simulink model "SoRo_Compliant_Demo_0906"  (R2023b)
settings: Solver=FixedStepAuto  StartTime=0.0  StopTime=inf  FixedStep=0.01  RelTol=1e-3
undefined symbols (not defined in the file): Down, Pull
libraries: simulink x50, speedgoatlib_IO691 x20, canmsglib x19, slpidlib x12, dspfdesign x6
(part 2 of 3)

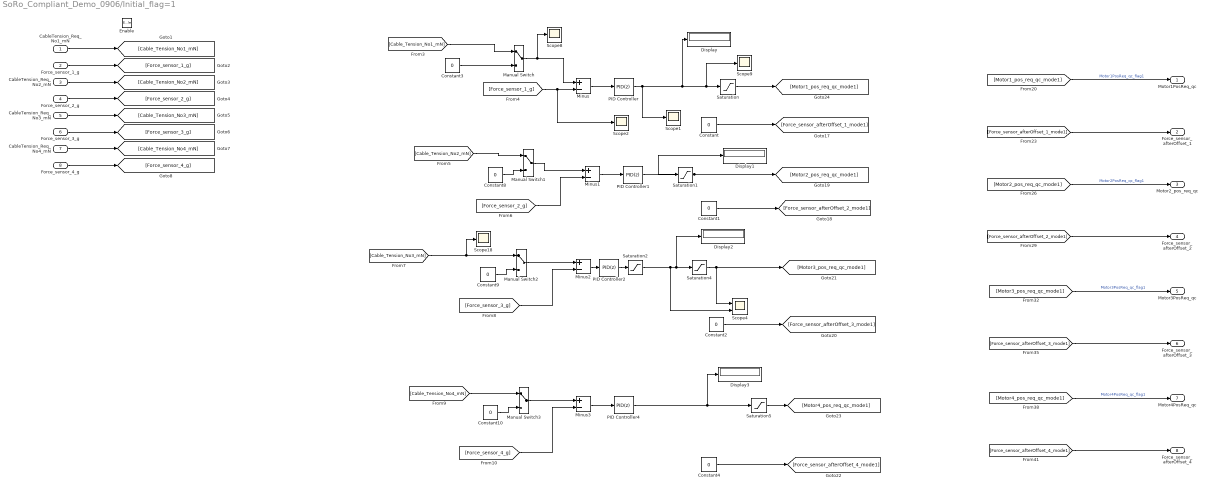
== system SoRo_Compliant_Demo_0906/Initial_flag=1 ==
  CableTension_Req_No1_mN : Inport
  Force_sensor_1_g : Inport  Port=2
  CableTension_Req_No2_mN : Inport  Port=3
  Force_sensor_2_g : Inport  Port=4
  CableTension_Req_No3_mN : Inport  Port=5
  Force_sensor_3_g : Inport  Port=6
  CableTension_Req_No4_mN : Inport  Port=7
  Force_sensor_4_g : Inport  Port=8
  Enable : EnablePort
  Constant{,1..2,4} (4 alike) : Constant  Value=0
  Constant{3,8..10} (4 alike) : Constant  Value=0  SampleTime=0.01
  Display{,1..3} (4 alike) : Display
  Manual Switch{,1..3} (4 alike) : ManualSwitch
  Minus{,1..3} (4 alike) : Sum  Inputs=+-
  PID Controller{,1..2,4} (4 alike) : slpidlib/PID Controller  Controller=PID  Form=Parallel  TimeDomain=Discrete-time  UseExternalTs=off  SampleTime=-1  IntegratorMethod=Forward Euler  FilterMethod=Forward Euler  ControllerParametersSource=internal  P=0.08  I=0.004  UseKiTs=off  D=0  N=100  UseFilter=on  TunerSelectOption=Transfer Function Based (PID Tuner App)  InitialConditionSource=internal  InitialConditionForIntegrator=0  InitialConditionForFilter=0  DifferentiatorICPrevScaledInput=0  ExternalReset=none  TrackingMode=off  Kt=1  LimitOutput=off  SatLimitsSource=internal  UpperSaturationLimit=inf  LowerSaturationLimit=-inf  LinearizeAsGain=on  AntiWindupMode=none  Kb=1  LimitIntegrator=off  UpperIntegratorSaturationLimit=inf  LowerIntegratorSaturationLimit=-inf  POutMin=[]  POutMax=[]  IOutMin=[]  IOutMax=[]  DOutMin=[]  DOutMax=[]  NOutMin=[]  NOutMax=[]  SumOutMin=[]  SumOutMax=[]  SaturationOutMin=[]  SaturationOutMax=[]  PParamMin=[]  PParamMax=[]  IParamMin=[]  IParamMax=[]  DParamMin=[]  DParamMax=[]  NParamMin=[]  NParamMax=[]  KbParamMin=[]  KbParamMax=[]  KtParamMin=[]  KtParamMax=[]  KbOutMin=[]  KbOutMax=[]  KtOutMin=[]  KtOutMax=[]  IntegratorOutMin=[]  IntegratorOutMax=[]  FilterOutMin=[]  FilterOutMax=[]  SumI1OutMin=[]  SumI1OutMax=[]  SumI2OutMin=[]  SumI2OutMax=[]  SumI3OutMin=[]  SumI3OutMax=[]  SumI4OutMin=[]  SumI4OutMax=[]  SumDOutMin=[]  SumDOutMax=[]  DifferentiatorOutMin=[]  DifferentiatorOutMax=[]  FilterDiffOutCoefMin=[]  FilterDiffOutCoefMax=[]  ReciprocalOutMin=[]  ReciprocalOutMax=[]  SumDenOutMin=[]  SumDenOutMax=[]  SumNumOutMin=[]  SumNumOutMax=[]  DivideOutMin=[]  DivideOutMax=[]  UdiffTsProdOutMin=[]  UdiffTsProdOutMax=[]  NTsProdOutMin=[]  NTsProdOutMax=[]  UintegralTsProdOutMin=[]  UintegralTsProdOutMax=[]  UngainTsProdOutMin=[]  UngainTsProdOutMax=[]  ClampingZeroOutDataTypeStr=Inherit: Inherit via back propagation  ClampingZeroOutMin=[]  ClampingZeroOutMax=[]  FilterDenConstantOutDataTypeStr=Inherit: Inherit via back propagation  FilterDenConstantOutMin=[]  FilterDenConstantOutMax=[]  PCopyOutDataTypeStr=Inherit: Inherit via back propagation  PCopyOutMin=[]  PCopyOutMax=[]  NCopyOutDataTypeStr=Inherit: Inherit via back propagation  NCopyOutMin=[]  NCopyOutMax=[]  IntegratorContinuousStateAttributes=''  IntegratorStateMustResolveToSignalObject=off  IntegratorRTWStateStorageClass=Auto  FilterContinuousStateAttributes=''  FilterStateMustResolveToSignalObject=off  FilterRTWStateStorageClass=Auto  ParallelPVariant=InternalParameters  IdealPVariant=Disabled  IVariant=InternalParameters  DVariant=InternalParameters  IntegratorVariant=Discrete  SatVariant=Disabled  AWVariant=Passthrough  PCopyVariant=Disabled  TRVariant=Disabled  FdbkBlocksVariant=Forward  IdealPFdbkVariant=Disabled  SatFdbkVariant=Disabled  DerivativeFilterVariant=ForwardEulerFilter  NVariant=InternalParameters  NCopyVariant=Disabled  FilterICVariant=InternalICsFilter  IntegratorICVariant=InternalICs  ExternalResetVariant=Disabled  TRSumVariant=Passthrough  SumFdbkVariant=Disabled  SumVariant=Sum_PID  TsampFilterVariant=InternalTs  TsampNgainVariant=Passthrough  TsampIntegralVariant=Disabled_SignalSpec  ExternalSaturationOutDataTypeStr=Inherit: Same as second input
  Saturation{,1,4..5} (4 alike) : Saturate  UpperLimit=3000  LowerLimit=-3000
  Saturation2 : Saturate  UpperLimit=400  LowerLimit=-400
  Scope{1..2,8..9,18} (5 alike) : Scope
  Scope4 : Scope  NumInputPorts=2
  Motor1PosReq_qc : Outport
  Force_sensor_afterOffset_1 : Outport  Port=2
  Motor2_pos_req_qc : Outport  Port=3
  Force_sensor_afterOffset_2 : Outport  Port=4
  Motor3PosReq_qc : Outport  Port=5
  Force_sensor_afterOffset_3 : Outport  Port=6
  Motor4PosReq_qc : Outport  Port=7
  Force_sensor_afterOffset_4 : Outport  Port=8
  wires:
  [Force_sensor_afterOffset_4_mode1] -> Force_sensor_afterOffset_4/1
  [Cable_Tension_No1_mN] -> Manual Switch/1
  [Cable_Tension_No4_mN] -> Manual Switch3/1
  Saturation/1 -> [Motor1_pos_req_qc_mode1]
  Constant1/1 -> [Force_sensor_afterOffset_2_mode1]
  [Force_sensor_afterOffset_2_mode1] -> Force_sensor_afterOffset_2/1
  PID Controller4/1 -> Display3/1, Saturation5/1
  PID Controller2/1 -> Saturation2/1
  Manual Switch2/1 -> Minus2/1
  [Cable_Tension_No3_mN] -> Scope18/1, Manual Switch2/1
  PID Controller/1 -> Display/1, Scope9/1, Saturation/1, Scope1/1
  Constant10/1 -> Manual Switch3/2
  Manual Switch3/1 -> Minus3/1
  Manual Switch/1 -> Scope8/1, Minus/1
  Manual Switch1/1 -> Minus1/1
  [Force_sensor_4_g] -> Minus3/2
  [Force_sensor_1_g] -> Scope2/1, Minus/2
  Constant4/1 -> [Force_sensor_afterOffset_4_mode1]
  Constant8/1 -> Manual Switch1/2
  [Cable_Tension_No2_mN] -> Manual Switch1/1
  Constant9/1 -> Manual Switch2/2
  [Force_sensor_2_g] -> Minus1/2
  CableTension_Req_No2_mN/1 -> [Cable_Tension_No2_mN]
  Minus1/1 -> PID Controller1/1
  CableTension_Req_No3_mN/1 -> [Cable_Tension_No3_mN]
  Saturation4/1 -> Scope4/1, [Motor3_pos_req_qc_mode1]
  PID Controller1/1 -> Saturation1/1
  [Force_sensor_afterOffset_3_mode1] -> Force_sensor_afterOffset_3/1
  Minus2/1 -> PID Controller2/1
  Minus/1 -> PID Controller/1
  Force_sensor_3_g/1 -> [Force_sensor_3_g]
  Minus3/1 -> PID Controller4/1
  Saturation2/1 -> Display2/1, Saturation4/1, Scope4/2
  Force_sensor_4_g/1 -> [Force_sensor_4_g]
  CableTension_Req_No4_mN/1 -> [Cable_Tension_No4_mN]
  [Motor4_pos_req_qc_mode1] -> Motor4PosReq_qc/1  "Motor4PosReq_qc_flag1"
  CableTension_Req_No1_mN/1 -> [Cable_Tension_No1_mN]
  Force_sensor_2_g/1 -> [Force_sensor_2_g]
  [Force_sensor_3_g] -> Minus2/2
  [Motor2_pos_req_qc_mode1] -> Motor2_pos_req_qc/1  "Motor2PosReq_qc_flag1"
  Force_sensor_1_g/1 -> [Force_sensor_1_g]
  [Motor3_pos_req_qc_mode1] -> Motor3PosReq_qc/1  "Motor3PosReq_qc_flag1"
  Constant2/1 -> [Force_sensor_afterOffset_3_mode1]
  [Motor1_pos_req_qc_mode1] -> Motor1PosReq_qc/1  "Motor1PosReq_qc_flag1"
  Saturation1/1 -> [Motor2_pos_req_qc_mode1], Display1/1
  Constant3/1 -> Manual Switch/2
  Constant/1 -> [Force_sensor_afterOffset_1_mode1]
  [Force_sensor_afterOffset_1_mode1] -> Force_sensor_afterOffset_1/1
  Saturation5/1 -> [Motor4_pos_req_qc_mode1]

== system SoRo_Compliant_Demo_0906/Subsystem ==
  Channel4 : Inport
  Enable : EnablePort
  " " : Constant  Value=5
  Gain4 : Gain  Gain=0.009
  MATLAB Function4 : MATLAB Function  TreatAsAtomicUnit=on
  MATLAB Function5 : MATLAB Function  TreatAsAtomicUnit=on
  Memory1 : Memory
  Minus2 : Sum  Inputs=+-
  Output Value at Neutral Position : Constant  Value=1000
  Scope{,1..3} (4 alike) : Scope
  Motor5PosReq_qc : Outport
  wires:
  Output Value at Neutral Position/1 -> Minus2/2
  MATLAB Function5/1(y) -> Scope1/1, Minus2/1
  Channel4/1 -> MATLAB Function5/1(u)
  " "/1 -> MATLAB Function5/2(threshold)
  Gain4/1 -> Scope3/1, MATLAB Function4/2(inc)
  Minus2/1 -> Scope2/1, Gain4/1
  Memory1/1 -> MATLAB Function4/1(otpt_last)
  MATLAB Function4/1(y) -> Scope/1, Memory1/1, Motor5PosReq_qc/1  "Motor5PosReq_qc"

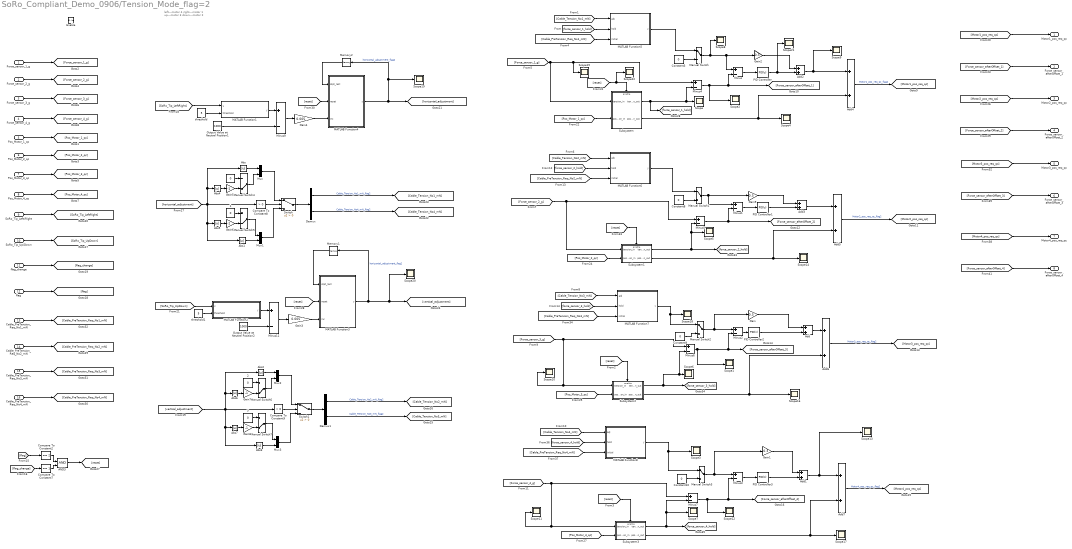
== system SoRo_Compliant_Demo_0906/Tension_Mode_flag=2 ==
  note: left---motor 4
      | right---motor 1
      | up---motor 3
      | down---motor 2
  Force_sensor_1_g : Inport
  Force_sensor_2_g : Inport  Port=2
  Force_sensor_3_g : Inport  Port=3
  Force_sensor_4_g : Inport  Port=4
  Pos_Motor_1_qc : Inport  Port=5
  Pos_Motor_2_qc : Inport  Port=6
  Pos_Motor_3_qc : Inport  Port=7
  Pos_Motor_4_qc : Inport  Port=8
  SoRo_Tip_Left/Right : Inport  Port=9
  SoRo_Tip_Up/Down : Inport  Port=10
  flag_change : Inport  Port=11
  flag : Inport  Port=12
  Cable_PreTension_Req_No1_mN : Inport  Port=13
  Cable_PreTension_Req_No2_mN : Inport  Port=14
  Cable_PreTension_Req_No3_mN : Inport  Port=15
  Cable_PreTension_Req_No4_mN : Inport  Port=16
  Enable : EnablePort
   {,1..3} (4 alike) : Constant  Value=0
  AND3 : Logic  IconShape=distinctive  AllPortsSameDT=off  OutDataTypeStr=boolean
  Abs{,1..7} (8 alike) : Abs  SaturateOnIntegerOverflow=off
  Add{,1..7} (8 alike) : Sum
  Compare To Constant2 : simulink/Logic and Bit Operations/Compare To Constant  relop===  const=2  OutDataTypeStr=boolean
  Compare To Constant7 : simulink/Logic and Bit Operations/Compare To Constant  relop===  const=1  OutDataTypeStr=boolean
  Compare To Constant8 : simulink/Logic and Bit Operations/Compare To Constant  relop=>  const=0  OutDataTypeStr=boolean
  Compare To Constant9 : simulink/Logic and Bit Operations/Compare To Constant  relop=>  const=0  OutDataTypeStr=boolean
  Constant{3,8..10} (4 alike) : Constant  Value=0  SampleTime=0.01
  Demux : Demux  Outputs=2
  Demux1 : Demux  Outputs=2
  Gain{,1..2,9} (4 alike) : Gain  Gain=0.3
  Gain3 : Gain  Gain=0.005
  Gain4 : Gain  Gain=0.005
  Gain{5..8} (4 alike) : Gain  Gain=-1
  MATLAB Function1 : MATLAB Function  TreatAsAtomicUnit=on
  MATLAB Function2 : MATLAB Function  TreatAsAtomicUnit=on
  MATLAB Function3 : MATLAB Function  TreatAsAtomicUnit=on
  MATLAB Function4 : MATLAB Function  TreatAsAtomicUnit=on
  MATLAB Function5 : MATLAB Function  TreatAsAtomicUnit=on
  MATLAB Function6 : MATLAB Function  TreatAsAtomicUnit=on
  MATLAB Function7 : MATLAB Function  TreatAsAtomicUnit=on
  MATLAB Function8 : MATLAB Function  TreatAsAtomicUnit=on
  Manual Switch{,1..3} (4 alike) : ManualSwitch
  Manual Switch{4..7} (4 alike) : ManualSwitch  CurrentSetting=0
  Memory1 : Memory
  Memory2 : Memory
  Minus{,1..7,9,11} (10 alike) : Sum  Inputs=+-
  Mux{,1..3} (4 alike) : Mux  Inputs=2
  Output Value at Neutral Position1 : Constant  Value=1000
  Output Value at Neutral Position2 : Constant  Value=1000
  PID Controller{,1..3} (4 alike) : slpidlib/PID Controller  Controller=PID  Form=Parallel  TimeDomain=Discrete-time  UseExternalTs=off  SampleTime=-1  IntegratorMethod=Forward Euler  FilterMethod=Forward Euler  ControllerParametersSource=internal  P=0.1  I=0  UseKiTs=off  D=0  N=100  UseFilter=on  TunerSelectOption=Transfer Function Based (PID Tuner App)  InitialConditionSource=internal  InitialConditionForIntegrator=0  InitialConditionForFilter=0  DifferentiatorICPrevScaledInput=0  ExternalReset=none  TrackingMode=off  Kt=1  LimitOutput=off  SatLimitsSource=internal  UpperSaturationLimit=inf  LowerSaturationLimit=-inf  LinearizeAsGain=on  AntiWindupMode=none  Kb=1  LimitIntegrator=off  UpperIntegratorSaturationLimit=inf  LowerIntegratorSaturationLimit=-inf  POutMin=[]  POutMax=[]  IOutMin=[]  IOutMax=[]  DOutMin=[]  DOutMax=[]  NOutMin=[]  NOutMax=[]  SumOutMin=[]  SumOutMax=[]  SaturationOutMin=[]  SaturationOutMax=[]  PParamMin=[]  PParamMax=[]  IParamMin=[]  IParamMax=[]  DParamMin=[]  DParamMax=[]  NParamMin=[]  NParamMax=[]  KbParamMin=[]  KbParamMax=[]  KtParamMin=[]  KtParamMax=[]  KbOutMin=[]  KbOutMax=[]  KtOutMin=[]  KtOutMax=[]  IntegratorOutMin=[]  IntegratorOutMax=[]  FilterOutMin=[]  FilterOutMax=[]  SumI1OutMin=[]  SumI1OutMax=[]  SumI2OutMin=[]  SumI2OutMax=[]  SumI3OutMin=[]  SumI3OutMax=[]  SumI4OutMin=[]  SumI4OutMax=[]  SumDOutMin=[]  SumDOutMax=[]  DifferentiatorOutMin=[]  DifferentiatorOutMax=[]  FilterDiffOutCoefMin=[]  FilterDiffOutCoefMax=[]  ReciprocalOutMin=[]  ReciprocalOutMax=[]  SumDenOutMin=[]  SumDenOutMax=[]  SumNumOutMin=[]  SumNumOutMax=[]  DivideOutMin=[]  DivideOutMax=[]  UdiffTsProdOutMin=[]  UdiffTsProdOutMax=[]  NTsProdOutMin=[]  NTsProdOutMax=[]  UintegralTsProdOutMin=[]  UintegralTsProdOutMax=[]  UngainTsProdOutMin=[]  UngainTsProdOutMax=[]  ClampingZeroOutDataTypeStr=Inherit: Inherit via back propagation  ClampingZeroOutMin=[]  ClampingZeroOutMax=[]  FilterDenConstantOutDataTypeStr=Inherit: Inherit via back propagation  FilterDenConstantOutMin=[]  FilterDenConstantOutMax=[]  PCopyOutDataTypeStr=Inherit: Inherit via back propagation  PCopyOutMin=[]  PCopyOutMax=[]  NCopyOutDataTypeStr=Inherit: Inherit via back propagation  NCopyOutMin=[]  NCopyOutMax=[]  IntegratorContinuousStateAttributes=''  IntegratorStateMustResolveToSignalObject=off  IntegratorRTWStateStorageClass=Auto  FilterContinuousStateAttributes=''  FilterStateMustResolveToSignalObject=off  FilterRTWStateStorageClass=Auto  ParallelPVariant=InternalParameters  IdealPVariant=Disabled  IVariant=InternalParameters  DVariant=InternalParameters  IntegratorVariant=Discrete  SatVariant=Disabled  AWVariant=Passthrough  PCopyVariant=Disabled  TRVariant=Disabled  FdbkBlocksVariant=Forward  IdealPFdbkVariant=Disabled  SatFdbkVariant=Disabled  DerivativeFilterVariant=ForwardEulerFilter  NVariant=InternalParameters  NCopyVariant=Disabled  FilterICVariant=InternalICsFilter  IntegratorICVariant=InternalICs  ExternalResetVariant=Disabled  TRSumVariant=Passthrough  SumFdbkVariant=Disabled  SumVariant=Sum_PID  TsampFilterVariant=InternalTs  TsampNgainVariant=Passthrough  TsampIntegralVariant=Disabled_SignalSpec  ExternalSaturationOutDataTypeStr=Inherit: Same as second input
  Scope{,1..22} (23 alike) : Scope
  Subsystem : Subsystem
  Subsystem1 : Subsystem
  Subsystem2 : Subsystem
  Subsystem3 : Subsystem
  Switch : Switch  Criteria=u2 > Threshold  SaturateOnIntegerOverflow=off  InputSameDT=off
  Switch1 : Switch  Criteria=u2 > Threshold  SaturateOnIntegerOverflow=off  InputSameDT=off
  threshold : Constant  Value=5
  threshold1 : Constant  Value=5
  Motor1_pos_req_qc : Outport
  Force_sensor_afterOffset_1 : Outport  Port=2
  Motor2_pos_req_qc : Outport  Port=3
  Force_sensor_afterOffset_2 : Outport  Port=4
  Motor3_pos_req_qc : Outport  Port=5
  Force_sensor_afterOffset_3 : Outport  Port=6
  Motor4_pos_req_qc : Outport  Port=7
  Force_sensor_afterOffset_4 : Outport  Port=8
  wires:
  [Force_sensor_1_g] -> Minus4/1, Scope15/1, Subsystem/1(tension_in)
  [Force_sensor_afterOffset_3] -> Force_sensor_afterOffset_3/1
  [Motor4_pos_req_qc] -> Motor4_pos_req_qc/1
  [Motor1_pos_req_qc] -> Motor1_pos_req_qc/1
  [Force_sensor_afterOffset_4] -> Force_sensor_afterOffset_4/1
  Constant9/1 -> Manual Switch2/2
  Subsystem2/1(tension_out) -> Minus6/2, Scope6/1, [force_sensor_3_hold]
  Minus/1 -> PID Controller/1
  Constant8/1 -> Manual Switch1/2
  [Motor3_pos_req_qc] -> Motor3_pos_req_qc/1
  Add1/1 -> Add7/1, Scope13/1
  Minus1/1 -> PID Controller1/1
  Subsystem3/1(tension_out) -> Scope7/1, Minus7/2, [force_sensor_4_hold]
  Minus7/1 -> Scope12/1, [Force_sensor_afterOffset_4], Minus3/2
  Manual Switch3/1 -> Minus3/1, Gain1/1
  [reset] -> Subsystem1/Enable
  PID Controller2/1 -> Add/2
  Minus5/1 -> [Force_sensor_afterOffset_2], Minus1/2
  Minus6/1 -> Scope1/1, [Force_sensor_afterOffset_3], Minus2/2
  Minus3/1 -> PID Controller3/1
  [Force_sensor_3_g] -> Minus6/1, Subsystem2/1(tension_in), Scope10/1
  Manual Switch/1 -> Minus/1, Gain2/1, Scope8/1
  Manual Switch2/1 -> Minus2/1, Gain/1
  Subsystem/1(tension_out) -> [force_sensor_1_hold], Scope/1, Minus4/2
  PID Controller/1 -> Scope21/1, Add2/2
  Constant10/1 -> Manual Switch3/2
  Subsystem1/1(tension_out) -> Minus5/2, Scope5/1, [force_sensor_2_hold]
  Gain1/1 -> Add1/1
  [reset] -> Scope22/1, Subsystem/Enable
  PID Controller3/1 -> Add1/2
  Gain/1 -> Add/1
  [Force_sensor_2_g] -> Subsystem1/1(tension_in), Minus5/1
  Force_sensor_4_g/1 -> [Force_sensor_4_g]
  [reset] -> Subsystem3/Enable
  Minus2/1 -> PID Controller2/1
  Constant3/1 -> Manual Switch/2
  Manual Switch1/1 -> Minus1/1, Gain9/1
  Force_sensor_3_g/1 -> [Force_sensor_3_g]
  Force_sensor_2_g/1 -> [Force_sensor_2_g]
  [reset] -> Subsystem2/Enable
  [Force_sensor_4_g] -> Minus7/1, Subsystem3/1(tension_in), Scope11/1
  [Force_sensor_afterOffset_1] -> Force_sensor_afterOffset_1/1
  [Motor2_pos_req_qc] -> Motor2_pos_req_qc/1
  Force_sensor_1_g/1 -> [Force_sensor_1_g]
  Gain2/1 -> Add2/1
  [Force_sensor_afterOffset_2] -> Force_sensor_afterOffset_2/1
  Add2/1 -> Add4/1, Scope9/1
  Minus4/1 -> Scope2/1, [Force_sensor_afterOffset_1], Minus/2
  SoRo_Tip_Left/Right/1 -> [SoRo_Tip_LeftRight]
  SoRo_Tip_Up/Down/1 -> [SoRo_Tip_UpDown]
  flag_change/1 -> [flag_change]
  flag/1 -> [flag]
  Gain4/1 -> MATLAB Function4/3(inc)
  Output Value at Neutral Position1/1 -> Minus9/2
  Minus9/1 -> Gain4/1
  [horizontal_adjustment] -> Compare To Constant8/1, Abs5/1, Abs1/1, Abs/1, Abs4/1
  Compare To Constant8/1 -> Switch/2
  Mux/1 -> Switch/1
  Switch/1 -> Demux/1
  Abs/1 -> Mux/1
  Mux1/1 -> Switch/3
  Manual Switch5/1 -> Mux1/1
  Abs1/1 -> Mux1/2
  Switch1/1 -> Demux1/1
  Gain3/1 -> MATLAB Function3/3(inc)
  Minus11/1 -> Gain3/1
  Output Value at Neutral Position2/1 -> Minus11/2
  MATLAB Function1/1(y) -> Minus9/1
  [SoRo_Tip_LeftRight] -> MATLAB Function1/1(u)
  threshold/1 -> MATLAB Function1/2(threshold)
  MATLAB Function2/1(y) -> Minus11/1
  [SoRo_Tip_UpDown] -> MATLAB Function2/1(u)
  threshold1/1 -> MATLAB Function2/2(threshold)
  Manual Switch4/1 -> Mux/2
  " "/1 -> Manual Switch4/1
  Abs4/1 -> Gain5/1
  Gain5/1 -> Manual Switch4/2
  Abs5/1 -> Gain6/1
  Gain6/1 -> Manual Switch5/2
  " 1"/1 -> Manual Switch5/1
  Manual Switch6/1 -> Mux2/2
  " 2"/1 -> Manual Switch6/1
  Gain8/1 -> Manual Switch7/2
  Abs7/1 -> Gain8/1
  Abs6/1 -> Gain7/1
  Gain7/1 -> Manual Switch6/2
  Abs3/1 -> Mux3/2
  Abs2/1 -> Mux2/1
  Mux3/1 -> Switch1/3
  Mux2/1 -> Switch1/1
  Compare To Constant9/1 -> Switch1/2
  Manual Switch7/1 -> Mux3/1
  [vertical_adjustment] -> Compare To Constant9/1, Abs7/1, Abs3/1, Abs2/1, Abs6/1
  " 3"/1 -> Manual Switch7/1
  PID Controller1/1 -> Add3/2
  Gain9/1 -> Add3/1
  Pos_Motor_1_qc/1 -> [Pos_Motor_1_qc]
  Pos_Motor_3_qc/1 -> [Pos_Motor_3_qc]
  Pos_Motor_4_qc/1 -> [Pos_Motor_4_qc]
  Pos_Motor_2_qc/1 -> [Pos_Motor_2_qc]
  [Pos_Motor_1_qc] -> Subsystem/2(position_in)
  Subsystem/2(position_out) -> Scope4/1, Add4/2
  Add4/1 -> [Motor1_pos_req_qc]  "Motor1_pos_req_qc_flag2"
  [Pos_Motor_2_qc] -> Subsystem1/2(position_in)
  Add3/1 -> Add5/1
  Add5/1 -> [Motor2_pos_req_qc]  "Motor2_pos_req_qc_flag2"
  [Pos_Motor_3_qc] -> Subsystem2/2(position_in)
  Add6/1 -> [Motor3_pos_req_qc]  "Motor3_pos_req_qc_flag2"
  Add/1 -> Add6/1
  [Pos_Motor_4_qc] -> Subsystem3/2(position_in)
  Add7/1 -> [Motor4_pos_req_qc]  "Motor4_pos_req_qc_flag2"
  MATLAB Function4/1(y) -> Memory2/1, Scope19/1, [horizontal_adjustment]  "horizontal_adjustment_flag2"
  MATLAB Function3/1(y) -> Memory1/1, Scope20/1, [vertical_adjustment]  "horizontal_adjustment_flag2"
  Compare To Constant2/1 -> AND3/1
  [flag] -> Compare To Constant2/1
  [flag_change] -> Compare To Constant7/1
  Compare To Constant7/1 -> AND3/2
  AND3/1 -> [reset]
  Memory2/1 -> MATLAB Function4/1(otpt_last)
  [reset] -> MATLAB Function4/2(reset)
  Memory1/1 -> MATLAB Function3/1(otpt_last)
  [reset] -> MATLAB Function3/2(reset)
  Subsystem1/2(position_out) -> Add5/2, Scope14/1
  Subsystem2/2(position_out) -> Scope16/1, Add6/2
  Subsystem3/2(position_out) -> Scope17/1, Add7/2
  Demux/1 -> [Cable_Tension_No1_mN]  "Cable_Tension_No1_mN_flag2"
  Demux/2 -> [Cable_Tension_No4_mN]  "Cable_Tension_No4_mN_flag2"
  Demux1/1 -> [Cable_Tension_No2_mN]  "Cable_Tension_No2_mN_flag2"
  Demux1/2 -> [Cable_Tension_No3_mN]  "Cable_Tension_No3_mN_flag2"
  MATLAB Function5/1(y) -> Manual Switch/1
  Cable_PreTension_Req_No2_mN/1 -> [Cable_PreTension_Req_No2_mN]
  Cable_PreTension_Req_No1_mN/1 -> [Cable_PreTension_Req_No1_mN]
  Cable_PreTension_Req_No4_mN/1 -> [Cable_PreTension_Req_No4_mN]
  Cable_PreTension_Req_No3_mN/1 -> [Cable_PreTension_Req_No3_mN]
  [force_sensor_1_hold] -> MATLAB Function5/2(hold)
  [Cable_Tension_No1_mN] -> MATLAB Function5/1(adj)
  [Cable_PreTension_Req_No1_mN] -> MATLAB Function5/3(initial)
  MATLAB Function6/1(y) -> Manual Switch1/1
  [Cable_Tension_No2_mN] -> MATLAB Function6/1(adj)
  [force_sensor_2_hold] -> MATLAB Function6/2(hold)
  [Cable_PreTension_Req_No2_mN] -> MATLAB Function6/3(initial)
  [force_sensor_3_hold] -> MATLAB Function7/2(hold)
  [Cable_PreTension_Req_No3_mN] -> MATLAB Function7/3(initial)
  [Cable_Tension_No3_mN] -> MATLAB Function7/1(adj)
  MATLAB Function7/1(y) -> Scope18/1, Manual Switch2/1
  [Cable_Tension_No4_mN] -> MATLAB Function8/1(adj)
  MATLAB Function8/1(y) -> Scope3/1, Manual Switch3/1
  [force_sensor_4_hold] -> MATLAB Function8/2(hold)
  [Cable_PreTension_Req_No4_mN] -> MATLAB Function8/3(initial)

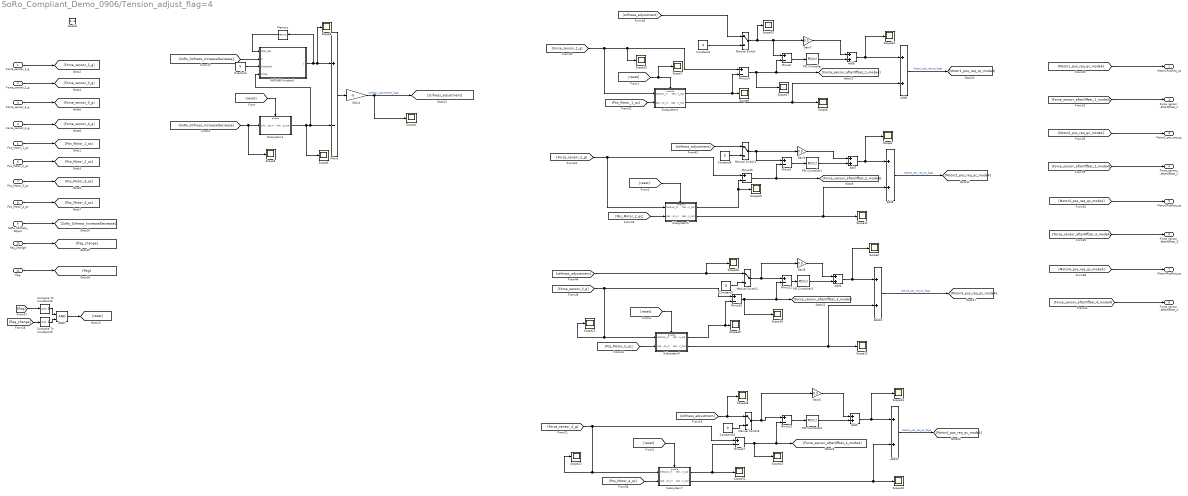
== system SoRo_Compliant_Demo_0906/Tension_adjust_flag=4 ==
  Force_sensor_1_g : Inport
  Force_sensor_2_g : Inport  Port=2
  Force_sensor_3_g : Inport  Port=3
  Force_sensor_4_g : Inport  Port=4
  Pos_Motor_1_qc : Inport  Port=5
  Pos_Motor_2_qc : Inport  Port=6
  Pos_Motor_3_qc : Inport  Port=7
  Pos_Motor_4_qc : Inport  Port=8
  SoRo_Stifness_Adjust : Inport  Port=9
  flag_change : Inport  Port=10
  flag : Inport  Port=11
  Enable : EnablePort  StatesWhenEnabling=reset
  AND7 : Logic  IconShape=distinctive  AllPortsSameDT=off  OutDataTypeStr=boolean
  Add{4..11} (8 alike) : Sum
  Compare To Constant10 : simulink/Logic and Bit Operations/Compare To Constant  relop===  const=4  OutDataTypeStr=boolean
  Compare To Constant15 : simulink/Logic and Bit Operations/Compare To Constant  relop===  const=1  OutDataTypeStr=boolean
  Constant{3,8..10} (4 alike) : Constant  Value=0  SampleTime=0.01
  Gain4 : Gain  Gain=-5
  Gain{5..7,9} (4 alike) : Gain  Gain=0.3
  MATLAB Function1 : MATLAB Function  TreatAsAtomicUnit=on
  Manual Switch{,1..3} (4 alike) : ManualSwitch
  Memory : Memory
  Minus{,2..3,12..17} (9 alike) : Sum  Inputs=+-
  PID Controller{,1..3} (4 alike) : slpidlib/PID Controller  Controller=PID  Form=Parallel  TimeDomain=Discrete-time  UseExternalTs=off  SampleTime=-1  IntegratorMethod=Forward Euler  FilterMethod=Forward Euler  ControllerParametersSource=internal  P=0.1  I=0  UseKiTs=off  D=0  N=100  UseFilter=on  TunerSelectOption=Transfer Function Based (PID Tuner App)  InitialConditionSource=internal  InitialConditionForIntegrator=0  InitialConditionForFilter=0  DifferentiatorICPrevScaledInput=0  ExternalReset=none  TrackingMode=off  Kt=1  LimitOutput=off  SatLimitsSource=internal  UpperSaturationLimit=inf  LowerSaturationLimit=-inf  LinearizeAsGain=on  AntiWindupMode=none  Kb=1  LimitIntegrator=off  UpperIntegratorSaturationLimit=inf  LowerIntegratorSaturationLimit=-inf  POutMin=[]  POutMax=[]  IOutMin=[]  IOutMax=[]  DOutMin=[]  DOutMax=[]  NOutMin=[]  NOutMax=[]  SumOutMin=[]  SumOutMax=[]  SaturationOutMin=[]  SaturationOutMax=[]  PParamMin=[]  PParamMax=[]  IParamMin=[]  IParamMax=[]  DParamMin=[]  DParamMax=[]  NParamMin=[]  NParamMax=[]  KbParamMin=[]  KbParamMax=[]  KtParamMin=[]  KtParamMax=[]  KbOutMin=[]  KbOutMax=[]  KtOutMin=[]  KtOutMax=[]  IntegratorOutMin=[]  IntegratorOutMax=[]  FilterOutMin=[]  FilterOutMax=[]  SumI1OutMin=[]  SumI1OutMax=[]  SumI2OutMin=[]  SumI2OutMax=[]  SumI3OutMin=[]  SumI3OutMax=[]  SumI4OutMin=[]  SumI4OutMax=[]  SumDOutMin=[]  SumDOutMax=[]  DifferentiatorOutMin=[]  DifferentiatorOutMax=[]  FilterDiffOutCoefMin=[]  FilterDiffOutCoefMax=[]  ReciprocalOutMin=[]  ReciprocalOutMax=[]  SumDenOutMin=[]  SumDenOutMax=[]  SumNumOutMin=[]  SumNumOutMax=[]  DivideOutMin=[]  DivideOutMax=[]  UdiffTsProdOutMin=[]  UdiffTsProdOutMax=[]  NTsProdOutMin=[]  NTsProdOutMax=[]  UintegralTsProdOutMin=[]  UintegralTsProdOutMax=[]  UngainTsProdOutMin=[]  UngainTsProdOutMax=[]  ClampingZeroOutDataTypeStr=Inherit: Inherit via back propagation  ClampingZeroOutMin=[]  ClampingZeroOutMax=[]  FilterDenConstantOutDataTypeStr=Inherit: Inherit via back propagation  FilterDenConstantOutMin=[]  FilterDenConstantOutMax=[]  PCopyOutDataTypeStr=Inherit: Inherit via back propagation  PCopyOutMin=[]  PCopyOutMax=[]  NCopyOutDataTypeStr=Inherit: Inherit via back propagation  NCopyOutMin=[]  NCopyOutMax=[]  IntegratorContinuousStateAttributes=''  IntegratorStateMustResolveToSignalObject=off  IntegratorRTWStateStorageClass=Auto  FilterContinuousStateAttributes=''  FilterStateMustResolveToSignalObject=off  FilterRTWStateStorageClass=Auto  ParallelPVariant=InternalParameters  IdealPVariant=Disabled  IVariant=InternalParameters  DVariant=InternalParameters  IntegratorVariant=Discrete  SatVariant=Disabled  AWVariant=Passthrough  PCopyVariant=Disabled  TRVariant=Disabled  FdbkBlocksVariant=Forward  IdealPFdbkVariant=Disabled  SatFdbkVariant=Disabled  DerivativeFilterVariant=ForwardEulerFilter  NVariant=InternalParameters  NCopyVariant=Disabled  FilterICVariant=InternalICsFilter  IntegratorICVariant=InternalICs  ExternalResetVariant=Disabled  TRSumVariant=Passthrough  SumFdbkVariant=Disabled  SumVariant=Sum_PID  TsampFilterVariant=InternalTs  TsampNgainVariant=Passthrough  TsampIntegralVariant=Disabled_SignalSpec  ExternalSaturationOutDataTypeStr=Inherit: Same as second input
  Scope{1..12,18,21..33} (26 alike) : Scope
  Subsystem1 : Subsystem
  Subsystem4 : Subsystem
  Subsystem5 : Subsystem
  Subsystem6 : Subsystem
  Subsystem7 : Subsystem
  threshold : Constant  Value=5
  Motor1PosReq_qc : Outport
  Force_sensor_afterOffset_1 : Outport  Port=2
  Motor2_pos_req_qc : Outport  Port=3
  Force_sensor_afterOffset_2 : Outport  Port=4
  Motor3PosReq_qc : Outport  Port=5
  Force_sensor_afterOffset_3 : Outport  Port=6
  Motor4PosReq_qc : Outport  Port=7
  Force_sensor_afterOffset_4 : Outport  Port=8
  wires:
  [Force_sensor_afterOffset_4_mode4] -> Force_sensor_afterOffset_4/1
  [Force_sensor_afterOffset_2_mode4] -> Force_sensor_afterOffset_2/1
  [Force_sensor_afterOffset_3_mode4] -> Force_sensor_afterOffset_3/1
  [Motor4_pos_req_qc_mode4] -> Motor4PosReq_qc/1
  [Motor2_pos_req_qc_mode4] -> Motor2_pos_req_qc/1
  [Motor3_pos_req_qc_mode4] -> Motor3PosReq_qc/1
  [Motor1_pos_req_qc_mode4] -> Motor1PosReq_qc/1
  [Force_sensor_afterOffset_1_mode4] -> Force_sensor_afterOffset_1/1
  Subsystem1/1(InitialSwitchValue_out) -> Scope3/1, MATLAB Function1/4(initial), Minus/2
  Minus/1 -> Gain4/1
  Gain4/1 -> [stifness_adjustment], Scope4/1  "stifness_adjustment_flag4"
  MATLAB Function1/1(y) -> Memory/1, Scope8/1, Minus/1
  [SoRo_Stifness_IncreaseDecrease] -> MATLAB Function1/2(u)
  threshold/1 -> MATLAB Function1/3(threshold)
  Pos_Motor_2_qc/1 -> [Pos_Motor_2_qc]
  Pos_Motor_4_qc/1 -> [Pos_Motor_4_qc]
  Pos_Motor_3_qc/1 -> [Pos_Motor_3_qc]
  Pos_Motor_1_qc/1 -> [Pos_Motor_1_qc]
  flag_change/1 -> [flag_change]
  Force_sensor_1_g/1 -> [Force_sensor_1_g]
  Force_sensor_4_g/1 -> [Force_sensor_4_g]
  Force_sensor_3_g/1 -> [Force_sensor_3_g]
  Force_sensor_2_g/1 -> [Force_sensor_2_g]
  SoRo_Stifness_Adjust/1 -> [SoRo_Stifness_IncreaseDecrease]
  flag/1 -> [flag]
  Subsystem5/1(tension_out) -> Minus15/2, Scope29/1
  [Pos_Motor_4_qc] -> Subsystem7/2(position_in)
  [reset] -> Subsystem7/Enable
  Add4/1 -> Scope2/1, Add10/1
  [Pos_Motor_2_qc] -> Subsystem5/2(position_in)
  [reset] -> Subsystem6/Enable
  Add7/1 -> Scope1/1, Add9/1
  [stifness_adjustment] -> Scope28/1, Manual Switch3/1
  Minus15/1 -> [Force_sensor_afterOffset_2_mode4], Minus3/2
  Gain7/1 -> Add6/1
  PID Controller3/1 -> Add5/2
  [stifness_adjustment] -> Scope26/1, Manual Switch2/1
  [reset] -> Scope7/1, Subsystem4/Enable
  Subsystem6/1(tension_out) -> Minus16/2, Scope30/1
  PID Controller/1 -> Add6/2
  Add5/1 -> Add11/1, Scope24/1
  PID Controller2/1 -> Add4/2
  Manual Switch2/1 -> Minus12/1, Gain5/1
  Subsystem4/1(tension_out) -> Minus14/2, Scope9/1
  Constant8/1 -> Manual Switch1/2
  [Force_sensor_1_g] -> Scope25/1, Minus14/1, Subsystem4/1(tension_in)
  Add10/1 -> [Motor3_pos_req_qc_mode4]  "Motor3_pos_req_qc_flag4"
  [Pos_Motor_1_qc] -> Subsystem4/2(position_in)
  [reset] -> Subsystem5/Enable
  Add11/1 -> [Motor4_pos_req_qc_mode4]  "Motor4_pos_req_qc_flag4"
  Subsystem7/1(tension_out) -> Scope31/1, Minus17/2
  Add9/1 -> [Motor2_pos_req_qc_mode4]  "Motor2_pos_req_qc_flag4"
  [Pos_Motor_3_qc] -> Subsystem6/2(position_in)
  Add8/1 -> [Motor1_pos_req_qc_mode4]  "Motor1_pos_req_qc_flag4"
  Minus14/1 -> Scope27/1, [Force_sensor_afterOffset_1_mode4], Minus2/2
  [Force_sensor_2_g] -> Subsystem5/1(tension_in), Minus15/1
  Manual Switch1/1 -> Minus3/1, Gain9/1
  [stifness_adjustment] -> Manual Switch/1
  Manual Switch/1 -> Minus2/1, Gain7/1, Scope32/1
  [Force_sensor_4_g] -> Minus17/1, Subsystem7/1(tension_in), Scope22/1
  PID Controller1/1 -> Add7/2
  Minus12/1 -> PID Controller2/1
  Minus16/1 -> Scope18/1, [Force_sensor_afterOffset_3_mode4], Minus12/2
  Minus17/1 -> Scope23/1, [Force_sensor_afterOffset_4_mode4], Minus13/2
  Subsystem4/2(position_out) -> Add8/2, Scope6/1
  Gain9/1 -> Add7/1
  Manual Switch3/1 -> Minus13/1, Gain6/1
  Add6/1 -> Add8/1, Scope33/1
  [Force_sensor_3_g] -> Minus16/1, Subsystem6/1(tension_in), Scope21/1
  Constant3/1 -> Manual Switch/2
  Gain5/1 -> Add4/1
  Constant9/1 -> Manual Switch2/2
  Minus3/1 -> PID Controller1/1
  Constant10/1 -> Manual Switch3/2
  Minus13/1 -> PID Controller3/1
  Gain6/1 -> Add5/1
  Minus2/1 -> PID Controller/1
  [stifness_adjustment] -> Manual Switch1/1
  [reset] -> Subsystem1/Enable
  [SoRo_Stifness_IncreaseDecrease] -> Scope5/1, Subsystem1/1(InitialSwitchValue_in)
  [flag] -> Compare To Constant10/1
  Compare To Constant10/1 -> AND7/1
  Compare To Constant15/1 -> AND7/2
  [flag_change] -> Compare To Constant15/1
  AND7/1 -> [reset]
  Memory/1 -> MATLAB Function1/1(otpt_last)
  Subsystem5/2(position_out) -> Scope11/1, Add9/2
  Subsystem6/2(position_out) -> Scope12/1, Add10/2
  Subsystem7/2(position_out) -> Add11/2, Scope10/1

== system SoRo_Compliant_Demo_0906/Transmit ==
  note: 驱动器复位
  End Test : Inport
  Input : Inport  Port=2
  Compare To Constant : simulink/Logic and Bit Operations/Compare To Constant  relop===  const=100  OutDataTypeStr=boolean
  Compare To Constant1 : simulink/Logic and Bit Operations/Compare To Constant  relop===  const=200  OutDataTypeStr=boolean
  Compare To Constant{2,4..6,8} (5 alike) : simulink/Logic and Bit Operations/Compare To Constant  relop=>=  const=300  OutDataTypeStr=boolean
  Compare To Constant3 : simulink/Logic and Bit Operations/Compare To Constant  relop===  const=1  OutDataTypeStr=boolean
  Compare To Constant33 : simulink/Logic and Bit Operations/Compare To Constant  relop===  const=250  OutDataTypeStr=boolean
  Constant : Constant
  Demux1 : Demux  Outputs=5
  Display{1..2,4,6,8} (5 alike) : Display
  Driver_Upload : Subsystem
  Gain{,1..3} (4 alike) : Gain  Gain=-1
  Mode Selection : Subsystem  ScheduleAs=Aperiodic partition  PartitionName=TEMP_PRECOMP_PARTITION_NAME_MessageTriggeredSubsystem
  PosSpdMode1 : Subsystem
  PosSpdMode2 : Subsystem
  PosSpdMode3 : Subsystem
  PosSpdMode4 : Subsystem
  PosSpdMode5 : Subsystem
  Rate Transition1 : RateTransition  OutPortSampleTime=1
  Reset : Subsystem
  Reset_Manually : Subsystem
  Scope{,1..4} (5 alike) : Scope
  Sum : Sum  Inputs=|++  InputSameDT=on  SaturateOnIntegerOverflow=on  OutDataTypeStr=Inherit: Same as first input
  Unit Delay1 : UnitDelay  SampleTime=-1  HasFrameUpgradeWarning=on
  wires:
  Compare To Constant/1 -> Reset/Enable
  Compare To Constant1/1 -> Scope2/1, Mode Selection/Enable
  Constant/1 -> Sum/1
  Unit Delay1/1 -> Sum/2
  Compare To Constant2/1 -> Display2/1, PosSpdMode1/Enable
  [End] -> Compare To Constant3/1
  Compare To Constant3/1 -> Rate Transition1/1
  Rate Transition1/1 -> Reset_Manually/Trigger, Reset_Manually/Enable
  Demux1/1 -> [PosCmdDrv1_qc]
  Demux1/3 -> Gain1/1
  Demux1/4 -> Gain2/1
  Input/1 -> Demux1/1
  Demux1/2 -> Gain/1
  End Test/1 -> [End]
  Compare To Constant4/1 -> Display4/1, PosSpdMode2/Enable
  Compare To Constant5/1 -> Display6/1, PosSpdMode3/Enable
  Compare To Constant6/1 -> Display8/1, PosSpdMode4/Enable
  [time] -> Compare To Constant4/1
  [time] -> Compare To Constant5/1
  [time] -> Compare To Constant6/1
  Compare To Constant33/1 -> Driver_Upload/Enable
  Sum/1 -> [time], Compare To Constant2/1, Compare To Constant33/1, Compare To Constant1/1, Unit Delay1/1, Compare To Constant/1
  Gain/1 -> [PosCmdDrv2_qc]
  Gain1/1 -> [PosCmdDrv3_qc]
  Gain2/1 -> [PosCmdDrv4_qc]
  [PosCmdDrv1_qc] -> PosSpdMode1/1(Inport2)
  [PosCmdDrv3_qc] -> Scope1/1, PosSpdMode3/1(Inport2)
  [PosCmdDrv2_qc] -> Scope/1, PosSpdMode2/1(Inport2)
  [PosCmdDrv4_qc] -> Scope3/1, PosSpdMode4/1(Inport2)
  Compare To Constant8/1 -> Display1/1, PosSpdMode5/Enable
  [PosCmdDrv5_qc] -> Scope4/1, PosSpdMode5/1(Inport2)
  [time] -> Compare To Constant8/1
  Demux1/5 -> Gain3/1
  Gain3/1 -> [PosCmdDrv5_qc]

== system SoRo_Compliant_Demo_0906/Displacement_mode_flag=3/Subsystem1 ==
  position_in : Inport
  Enable : EnablePort
  position_out : Outport
  wires:
  position_in/1 -> position_out/1

== system SoRo_Compliant_Demo_0906/Displacement_mode_flag=3/Subsystem2 ==
  position_in : Inport
  Enable : EnablePort
  position_out : Outport
  wires:
  position_in/1 -> position_out/1

== system SoRo_Compliant_Demo_0906/Displacement_mode_flag=3/Subsystem3 ==
  position_in : Inport
  Enable : EnablePort
  position_out : Outport
  wires:
  position_in/1 -> position_out/1

== system SoRo_Compliant_Demo_0906/Displacement_mode_flag=3/Subsystem5 ==
  position_in : Inport
  Enable : EnablePort
  position_out : Outport
  wires:
  position_in/1 -> position_out/1

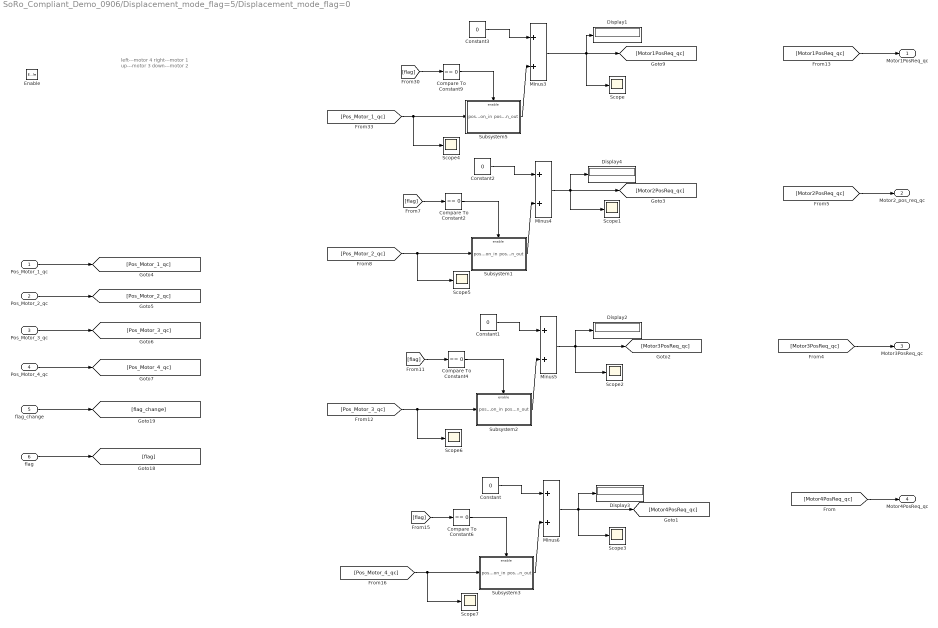
== system SoRo_Compliant_Demo_0906/Displacement_mode_flag=5/Displacement_mode_flag=0 ==
  note: left---motor 4
      | right---motor 1
      | up---motor 3
      | down---motor 2
  Pos_Motor_1_qc : Inport
  Pos_Motor_2_qc : Inport  Port=2
  Pos_Motor_3_qc : Inport  Port=3
  Pos_Motor_4_qc : Inport  Port=4
  flag_change : Inport  Port=5
  flag : Inport  Port=6
  Enable : EnablePort
  Compare To Constant{2,4,6,9} (4 alike) : simulink/Logic and Bit Operations/Compare To Constant  relop===  const=0  OutDataTypeStr=boolean
  Constant{,1..3} (4 alike) : Constant  Value=0
  Display{1..4} (4 alike) : Display
  Minus{3..6} (4 alike) : Sum
  Scope{,1..7} (8 alike) : Scope
  Subsystem1 : Subsystem
  Subsystem2 : Subsystem
  Subsystem3 : Subsystem
  Subsystem5 : Subsystem
  Motor1PosReq_qc : Outport
  Motor2_pos_req_qc : Outport  Port=2
  Motor3PosReq_qc : Outport  Port=3
  Motor4PosReq_qc : Outport  Port=4
  wires:
  Pos_Motor_4_qc/1 -> [Pos_Motor_4_qc]
  Pos_Motor_3_qc/1 -> [Pos_Motor_3_qc]
  Pos_Motor_2_qc/1 -> [Pos_Motor_2_qc]
  Pos_Motor_1_qc/1 -> [Pos_Motor_1_qc]
  flag/1 -> [flag]
  flag_change/1 -> [flag_change]
  [Pos_Motor_1_qc] -> Scope4/1, Subsystem5/1(position_in)
  [flag] -> Compare To Constant9/1
  Compare To Constant9/1 -> Subsystem5/Enable
  Constant3/1 -> Minus3/1
  Minus3/1 -> [Motor1PosReq_qc], Scope/1, Display1/1
  Subsystem5/1(position_out) -> Minus3/2
  Constant2/1 -> Minus4/1
  Compare To Constant2/1 -> Subsystem1/Enable
  [Pos_Motor_2_qc] -> Scope5/1, Subsystem1/1(position_in)
  Minus4/1 -> [Motor2PosReq_qc], Scope1/1, Display4/1
  Subsystem1/1(position_out) -> Minus4/2
  [flag] -> Compare To Constant2/1
  [flag] -> Compare To Constant4/1
  Subsystem2/1(position_out) -> Minus5/2
  Minus5/1 -> [Motor3PosReq_qc], Scope2/1, Display2/1
  Compare To Constant4/1 -> Subsystem2/Enable
  [Pos_Motor_3_qc] -> Scope6/1, Subsystem2/1(position_in)
  Constant1/1 -> Minus5/1
  [flag] -> Compare To Constant6/1
  Subsystem3/1(position_out) -> Minus6/2
  Minus6/1 -> [Motor4PosReq_qc], Scope3/1, Display3/1
  Compare To Constant6/1 -> Subsystem3/Enable
  [Pos_Motor_4_qc] -> Scope7/1, Subsystem3/1(position_in)
  Constant/1 -> Minus6/1
  [Motor4PosReq_qc] -> Motor4PosReq_qc/1
  [Motor3PosReq_qc] -> Motor3PosReq_qc/1
  [Motor2PosReq_qc] -> Motor2_pos_req_qc/1
  [Motor1PosReq_qc] -> Motor1PosReq_qc/1

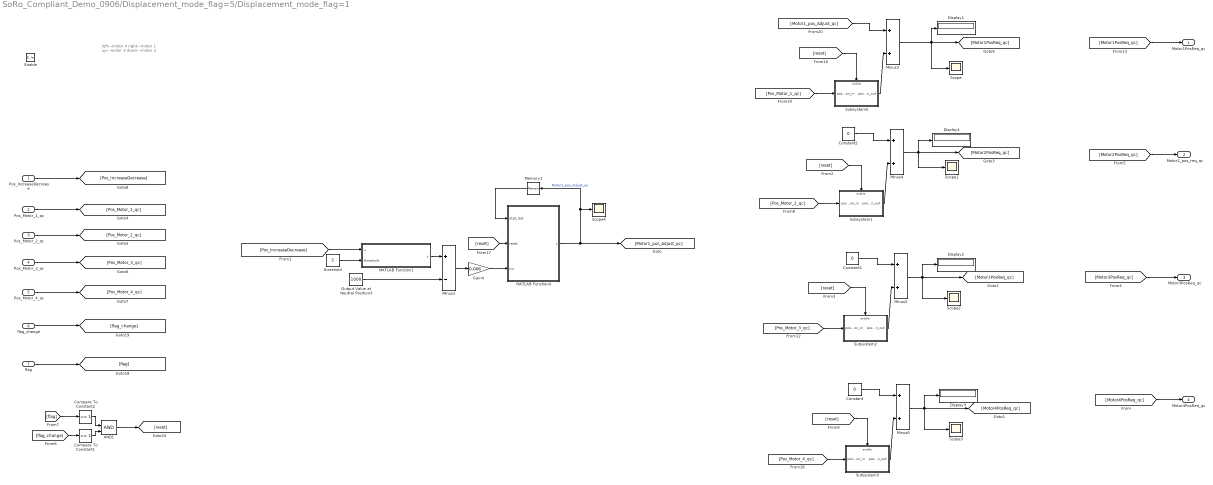
== system SoRo_Compliant_Demo_0906/Displacement_mode_flag=5/Displacement_mode_flag=1 ==
  note: left---motor 4
      | right---motor 1
      | up---motor 3
      | down---motor 2
  Pos_IncreaseDecrease : Inport
  Pos_Motor_1_qc : Inport  Port=2
  Pos_Motor_2_qc : Inport  Port=3
  Pos_Motor_3_qc : Inport  Port=4
  Pos_Motor_4_qc : Inport  Port=5
  flag_change : Inport  Port=6
  flag : Inport  Port=7
  Enable : EnablePort
  AND1 : Logic  IconShape=distinctive  AllPortsSameDT=off  OutDataTypeStr=boolean
  Compare To Constant1 : simulink/Logic and Bit Operations/Compare To Constant  relop===  const=1  OutDataTypeStr=boolean
  Compare To Constant2 : simulink/Logic and Bit Operations/Compare To Constant  relop===  const=1  OutDataTypeStr=boolean
  Constant : Constant  Value=0
  Constant1 : Constant  Value=0
  Constant2 : Constant  Value=0
  Display{1..4} (4 alike) : Display
  Gain4 : Gain  Gain=0.006
  MATLAB Function1 : MATLAB Function  TreatAsAtomicUnit=on
  MATLAB Function4 : MATLAB Function  TreatAsAtomicUnit=on
  Memory1 : Memory
  Minus2 : Sum  Inputs=+-
  Minus{3..6} (4 alike) : Sum
  Output Value at Neutral Position3 : Constant  Value=1000
  Scope{,1..4} (5 alike) : Scope
  Subsystem1 : Subsystem
  Subsystem2 : Subsystem
  Subsystem3 : Subsystem
  Subsystem5 : Subsystem
  threshold : Constant  Value=5
  Motor1PosReq_qc : Outport
  Motor2_pos_req_qc : Outport  Port=2
  Motor3PosReq_qc : Outport  Port=3
  Motor4PosReq_qc : Outport  Port=4
  wires:
  Minus2/1 -> Gain4/1
  [Pos_IncreaseDecrease] -> MATLAB Function1/1(u)
  MATLAB Function1/1(y) -> Minus2/1
  threshold/1 -> MATLAB Function1/2(threshold)
  Output Value at Neutral Position3/1 -> Minus2/2
  Pos_Motor_4_qc/1 -> [Pos_Motor_4_qc]
  Pos_Motor_3_qc/1 -> [Pos_Motor_3_qc]
  Pos_Motor_2_qc/1 -> [Pos_Motor_2_qc]
  Pos_Motor_1_qc/1 -> [Pos_Motor_1_qc]
  flag/1 -> [flag]
  flag_change/1 -> [flag_change]
  [Pos_Motor_1_qc] -> Subsystem5/1(position_in)
  [reset] -> Subsystem5/Enable
  [Motor1_pos_Adjust_qc] -> Minus3/1
  Minus3/1 -> [Motor1PosReq_qc], Scope/1, Display1/1
  Subsystem5/1(position_out) -> Minus3/2
  Constant2/1 -> Minus4/1
  [reset] -> Subsystem1/Enable
  [Pos_Motor_2_qc] -> Subsystem1/1(position_in)
  Minus4/1 -> [Motor2PosReq_qc], Scope1/1, Display4/1
  Subsystem1/1(position_out) -> Minus4/2
  Subsystem2/1(position_out) -> Minus5/2
  Minus5/1 -> [Motor3PosReq_qc], Scope2/1, Display2/1
  [reset] -> Subsystem2/Enable
  [Pos_Motor_3_qc] -> Subsystem2/1(position_in)
  Constant1/1 -> Minus5/1
  Subsystem3/1(position_out) -> Minus6/2
  Minus6/1 -> [Motor4PosReq_qc], Scope3/1, Display3/1
  [reset] -> Subsystem3/Enable
  [Pos_Motor_4_qc] -> Subsystem3/1(position_in)
  Constant/1 -> Minus6/1
  Gain4/1 -> MATLAB Function4/3(inc)
  Pos_IncreaseDecrease/1 -> [Pos_IncreaseDecrease]
  [Motor4PosReq_qc] -> Motor4PosReq_qc/1
  [Motor3PosReq_qc] -> Motor3PosReq_qc/1
  [Motor2PosReq_qc] -> Motor2_pos_req_qc/1
  [Motor1PosReq_qc] -> Motor1PosReq_qc/1
  [reset] -> MATLAB Function4/2(reset)
  Memory1/1 -> MATLAB Function4/1(otpt_last)
  MATLAB Function4/1(y) -> [Motor1_pos_Adjust_qc], Memory1/1, Scope4/1  "Motor1_pos_Adjust_qc"
  Compare To Constant1/1 -> AND1/2
  [flag_change] -> Compare To Constant1/1
  Compare To Constant2/1 -> AND1/1
  [flag] -> Compare To Constant2/1
  AND1/1 -> [reset]

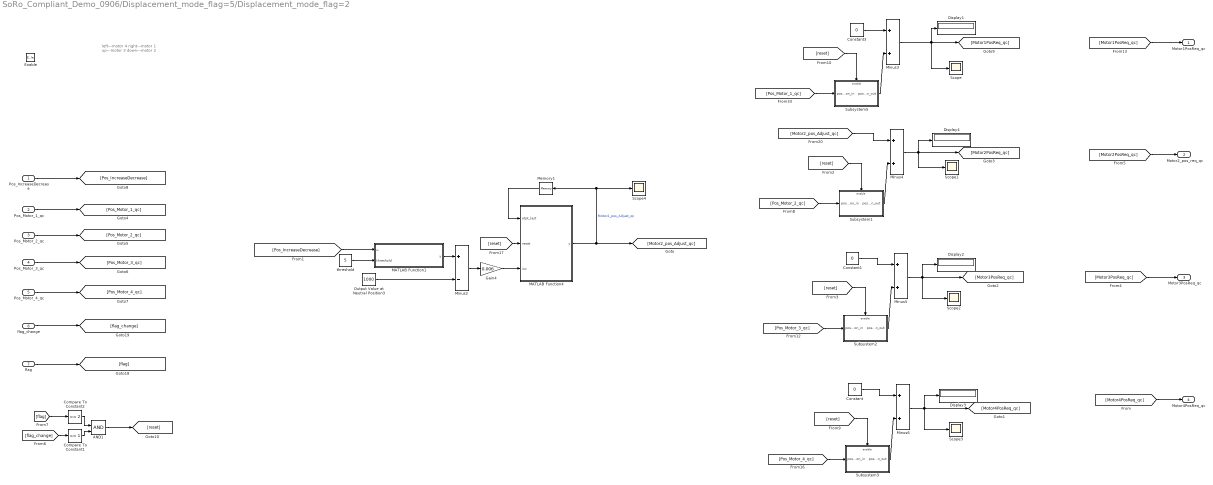
== system SoRo_Compliant_Demo_0906/Displacement_mode_flag=5/Displacement_mode_flag=2 ==
  note: left---motor 4
      | right---motor 1
      | up---motor 3
      | down---motor 2
  Pos_IncreaseDecrease : Inport
  Pos_Motor_1_qc : Inport  Port=2
  Pos_Motor_2_qc : Inport  Port=3
  Pos_Motor_3_qc : Inport  Port=4
  Pos_Motor_4_qc : Inport  Port=5
  flag_change : Inport  Port=6
  flag : Inport  Port=7
  Enable : EnablePort
  AND1 : Logic  IconShape=distinctive  AllPortsSameDT=off  OutDataTypeStr=boolean
  Compare To Constant1 : simulink/Logic and Bit Operations/Compare To Constant  relop===  const=1  OutDataTypeStr=boolean
  Compare To Constant2 : simulink/Logic and Bit Operations/Compare To Constant  relop===  const=2  OutDataTypeStr=boolean
  Constant : Constant  Value=0
  Constant1 : Constant  Value=0
  Constant3 : Constant  Value=0
  Display{1..4} (4 alike) : Display
  Gain4 : Gain  Gain=0.006
  MATLAB Function1 : MATLAB Function  TreatAsAtomicUnit=on
  MATLAB Function4 : MATLAB Function  TreatAsAtomicUnit=on
  Memory1 : Memory
  Minus2 : Sum  Inputs=+-
  Minus{3..6} (4 alike) : Sum
  Output Value at Neutral Position3 : Constant  Value=1000
  Scope{,1..4} (5 alike) : Scope
  Subsystem1 : Subsystem
  Subsystem2 : Subsystem
  Subsystem3 : Subsystem
  Subsystem5 : Subsystem
  threshold : Constant  Value=5
  Motor1PosReq_qc : Outport
  Motor2_pos_req_qc : Outport  Port=2
  Motor3PosReq_qc : Outport  Port=3
  Motor4PosReq_qc : Outport  Port=4
  wires:
  Minus2/1 -> Gain4/1
  [Pos_IncreaseDecrease] -> MATLAB Function1/1(u)
  MATLAB Function1/1(y) -> Minus2/1
  threshold/1 -> MATLAB Function1/2(threshold)
  Output Value at Neutral Position3/1 -> Minus2/2
  Pos_Motor_4_qc/1 -> [Pos_Motor_4_qc]
  Pos_Motor_3_qc/1 -> [Pos_Motor_3_qc]
  Pos_Motor_2_qc/1 -> [Pos_Motor_2_qc]
  Pos_Motor_1_qc/1 -> [Pos_Motor_1_qc]
  flag/1 -> [flag]
  flag_change/1 -> [flag_change]
  [Pos_Motor_1_qc] -> Subsystem5/1(position_in)
  [reset] -> Subsystem5/Enable
  Minus3/1 -> [Motor1PosReq_qc], Scope/1, Display1/1
  Subsystem5/1(position_out) -> Minus3/2
  [Motor2_pos_Adjust_qc] -> Minus4/1
  [reset] -> Subsystem1/Enable
  [Pos_Motor_2_qc] -> Subsystem1/1(position_in)
  Minus4/1 -> [Motor2PosReq_qc], Scope1/1, Display4/1
  Subsystem1/1(position_out) -> Minus4/2
  Subsystem2/1(position_out) -> Minus5/2
  Minus5/1 -> [Motor3PosReq_qc], Scope2/1, Display2/1
  [reset] -> Subsystem2/Enable
  [Pos_Motor_3_qc] -> Subsystem2/1(position_in)
  Constant1/1 -> Minus5/1
  Subsystem3/1(position_out) -> Minus6/2
  Minus6/1 -> [Motor4PosReq_qc], Scope3/1, Display3/1
  [reset] -> Subsystem3/Enable
  [Pos_Motor_4_qc] -> Subsystem3/1(position_in)
  Constant/1 -> Minus6/1
  Gain4/1 -> MATLAB Function4/3(inc)
  Pos_IncreaseDecrease/1 -> [Pos_IncreaseDecrease]
  [Motor4PosReq_qc] -> Motor4PosReq_qc/1
  [Motor3PosReq_qc] -> Motor3PosReq_qc/1
  [Motor2PosReq_qc] -> Motor2_pos_req_qc/1
  [Motor1PosReq_qc] -> Motor1PosReq_qc/1
  Constant3/1 -> Minus3/1
  Compare To Constant1/1 -> AND1/2
  [flag_change] -> Compare To Constant1/1
  Compare To Constant2/1 -> AND1/1
  [flag] -> Compare To Constant2/1
  AND1/1 -> [reset]
  [reset] -> MATLAB Function4/2(reset)
  Memory1/1 -> MATLAB Function4/1(otpt_last)
  MATLAB Function4/1(y) -> Scope4/1, Memory1/1, [Motor2_pos_Adjust_qc]  "Motor2_pos_Adjust_qc"

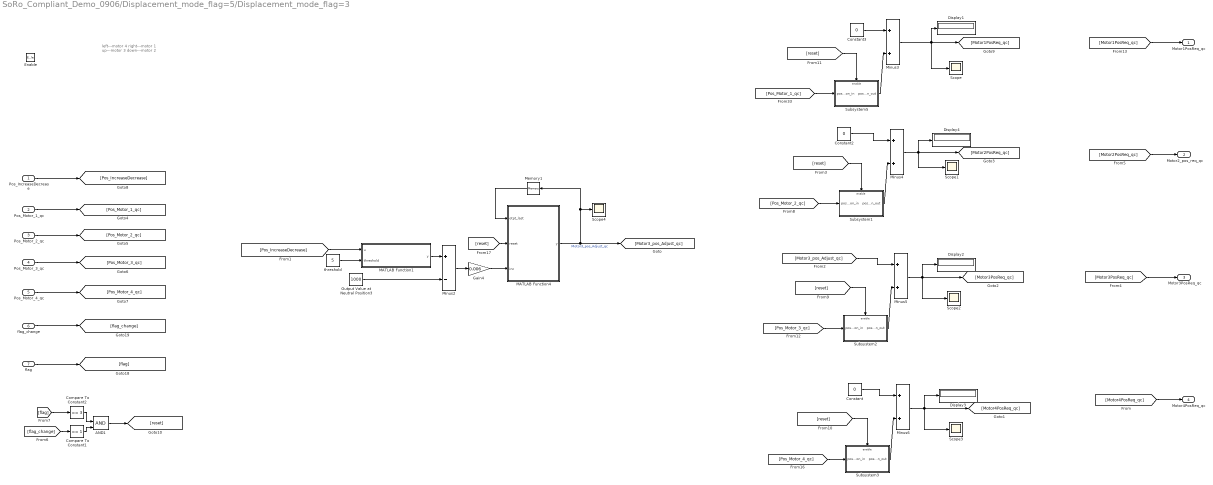
== system SoRo_Compliant_Demo_0906/Displacement_mode_flag=5/Displacement_mode_flag=3 ==
  note: left---motor 4
      | right---motor 1
      | up---motor 3
      | down---motor 2
  Pos_IncreaseDecrease : Inport
  Pos_Motor_1_qc : Inport  Port=2
  Pos_Motor_2_qc : Inport  Port=3
  Pos_Motor_3_qc : Inport  Port=4
  Pos_Motor_4_qc : Inport  Port=5
  flag_change : Inport  Port=6
  flag : Inport  Port=7
  Enable : EnablePort
  AND1 : Logic  IconShape=distinctive  AllPortsSameDT=off  OutDataTypeStr=boolean
  Compare To Constant1 : simulink/Logic and Bit Operations/Compare To Constant  relop===  const=1  OutDataTypeStr=boolean
  Compare To Constant2 : simulink/Logic and Bit Operations/Compare To Constant  relop===  const=3  OutDataTypeStr=boolean
  Constant : Constant  Value=0
  Constant2 : Constant  Value=0
  Constant3 : Constant  Value=0
  Display{1..4} (4 alike) : Display
  Gain4 : Gain  Gain=0.006
  MATLAB Function1 : MATLAB Function  TreatAsAtomicUnit=on
  MATLAB Function4 : MATLAB Function  TreatAsAtomicUnit=on
  Memory1 : Memory
  Minus2 : Sum  Inputs=+-
  Minus{3..6} (4 alike) : Sum
  Output Value at Neutral Position3 : Constant  Value=1000
  Scope{,1..4} (5 alike) : Scope
  Subsystem1 : Subsystem
  Subsystem2 : Subsystem
  Subsystem3 : Subsystem
  Subsystem5 : Subsystem
  threshold : Constant  Value=5
  Motor1PosReq_qc : Outport
  Motor2_pos_req_qc : Outport  Port=2
  Motor3PosReq_qc : Outport  Port=3
  Motor4PosReq_qc : Outport  Port=4
  wires:
  Minus2/1 -> Gain4/1
  [Pos_IncreaseDecrease] -> MATLAB Function1/1(u)
  MATLAB Function1/1(y) -> Minus2/1
  threshold/1 -> MATLAB Function1/2(threshold)
  Output Value at Neutral Position3/1 -> Minus2/2
  Pos_Motor_4_qc/1 -> [Pos_Motor_4_qc]
  Pos_Motor_3_qc/1 -> [Pos_Motor_3_qc]
  Pos_Motor_2_qc/1 -> [Pos_Motor_2_qc]
  Pos_Motor_1_qc/1 -> [Pos_Motor_1_qc]
  flag/1 -> [flag]
  flag_change/1 -> [flag_change]
  [Pos_Motor_1_qc] -> Subsystem5/1(position_in)
  [reset] -> Subsystem5/Enable
  Minus3/1 -> [Motor1PosReq_qc], Scope/1, Display1/1
  Subsystem5/1(position_out) -> Minus3/2
  Constant2/1 -> Minus4/1
  [reset] -> Subsystem1/Enable
  [Pos_Motor_2_qc] -> Subsystem1/1(position_in)
  Minus4/1 -> [Motor2PosReq_qc], Scope1/1, Display4/1
  Subsystem1/1(position_out) -> Minus4/2
  Subsystem2/1(position_out) -> Minus5/2
  Minus5/1 -> [Motor3PosReq_qc], Scope2/1, Display2/1
  [reset] -> Subsystem2/Enable
  [Pos_Motor_3_qc] -> Subsystem2/1(position_in)
  [Motor3_pos_Adjust_qc] -> Minus5/1
  Subsystem3/1(position_out) -> Minus6/2
  Minus6/1 -> [Motor4PosReq_qc], Scope3/1, Display3/1
  [reset] -> Subsystem3/Enable
  [Pos_Motor_4_qc] -> Subsystem3/1(position_in)
  Constant/1 -> Minus6/1
  Gain4/1 -> MATLAB Function4/3(inc)
  Pos_IncreaseDecrease/1 -> [Pos_IncreaseDecrease]
  [Motor4PosReq_qc] -> Motor4PosReq_qc/1
  [Motor3PosReq_qc] -> Motor3PosReq_qc/1
  [Motor2PosReq_qc] -> Motor2_pos_req_qc/1
  [Motor1PosReq_qc] -> Motor1PosReq_qc/1
  Constant3/1 -> Minus3/1
  Compare To Constant1/1 -> AND1/2
  [flag_change] -> Compare To Constant1/1
  [flag] -> Compare To Constant2/1
  Compare To Constant2/1 -> AND1/1
  AND1/1 -> [reset]
  [reset] -> MATLAB Function4/2(reset)
  Memory1/1 -> MATLAB Function4/1(otpt_last)
  MATLAB Function4/1(y) -> Scope4/1, Memory1/1, [Motor3_pos_Adjust_qc]  "Motor3_pos_Adjust_qc"

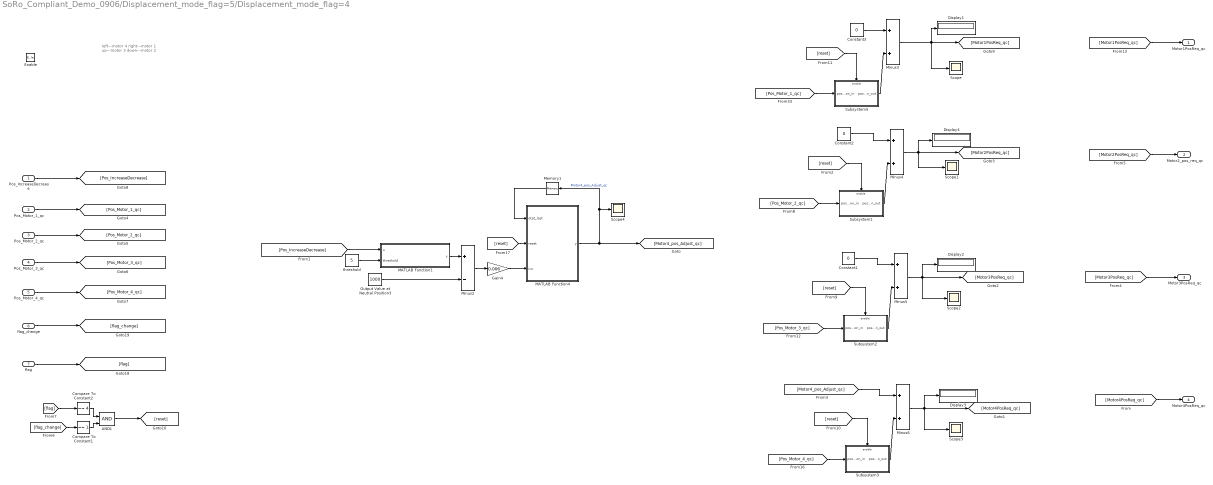
== system SoRo_Compliant_Demo_0906/Displacement_mode_flag=5/Displacement_mode_flag=4 ==
  note: left---motor 4
      | right---motor 1
      | up---motor 3
      | down---motor 2
  Pos_IncreaseDecrease : Inport
  Pos_Motor_1_qc : Inport  Port=2
  Pos_Motor_2_qc : Inport  Port=3
  Pos_Motor_3_qc : Inport  Port=4
  Pos_Motor_4_qc : Inport  Port=5
  flag_change : Inport  Port=6
  flag : Inport  Port=7
  Enable : EnablePort
  AND1 : Logic  IconShape=distinctive  AllPortsSameDT=off  OutDataTypeStr=boolean
  Compare To Constant1 : simulink/Logic and Bit Operations/Compare To Constant  relop===  const=1  OutDataTypeStr=boolean
  Compare To Constant2 : simulink/Logic and Bit Operations/Compare To Constant  relop===  const=4  OutDataTypeStr=boolean
  Constant1 : Constant  Value=0
  Constant2 : Constant  Value=0
  Constant3 : Constant  Value=0
  Display{1..4} (4 alike) : Display
  Gain4 : Gain  Gain=0.006
  MATLAB Function1 : MATLAB Function  TreatAsAtomicUnit=on
  MATLAB Function4 : MATLAB Function  TreatAsAtomicUnit=on
  Memory1 : Memory
  Minus2 : Sum  Inputs=+-
  Minus{3..6} (4 alike) : Sum
  Output Value at Neutral Position3 : Constant  Value=1000
  Scope{,1..4} (5 alike) : Scope
  Subsystem1 : Subsystem
  Subsystem2 : Subsystem
  Subsystem3 : Subsystem
  Subsystem5 : Subsystem
  threshold : Constant  Value=5
  Motor1PosReq_qc : Outport
  Motor2_pos_req_qc : Outport  Port=2
  Motor3PosReq_qc : Outport  Port=3
  Motor4PosReq_qc : Outport  Port=4
  wires:
  Constant3/1 -> Minus3/1
  [Motor1PosReq_qc] -> Motor1PosReq_qc/1
  [Motor2PosReq_qc] -> Motor2_pos_req_qc/1
  [Motor3PosReq_qc] -> Motor3PosReq_qc/1
  [Motor4PosReq_qc] -> Motor4PosReq_qc/1
  Pos_IncreaseDecrease/1 -> [Pos_IncreaseDecrease]
  Gain4/1 -> MATLAB Function4/3(inc)
  [Motor4_pos_Adjust_qc] -> Minus6/1
  [Pos_Motor_4_qc] -> Subsystem3/1(position_in)
  [reset] -> Subsystem3/Enable
  Minus6/1 -> Display3/1, Scope3/1, [Motor4PosReq_qc]
  Subsystem3/1(position_out) -> Minus6/2
  Constant1/1 -> Minus5/1
  [Pos_Motor_3_qc] -> Subsystem2/1(position_in)
  [reset] -> Subsystem2/Enable
  Minus5/1 -> Display2/1, Scope2/1, [Motor3PosReq_qc]
  Subsystem2/1(position_out) -> Minus5/2
  Subsystem1/1(position_out) -> Minus4/2
  Minus4/1 -> Display4/1, Scope1/1, [Motor2PosReq_qc]
  [Pos_Motor_2_qc] -> Subsystem1/1(position_in)
  [reset] -> Subsystem1/Enable
  Constant2/1 -> Minus4/1
  Subsystem5/1(position_out) -> Minus3/2
  Minus3/1 -> Display1/1, Scope/1, [Motor1PosReq_qc]
  [reset] -> Subsystem5/Enable
  [Pos_Motor_1_qc] -> Subsystem5/1(position_in)
  flag_change/1 -> [flag_change]
  flag/1 -> [flag]
  Pos_Motor_1_qc/1 -> [Pos_Motor_1_qc]
  Pos_Motor_2_qc/1 -> [Pos_Motor_2_qc]
  Pos_Motor_3_qc/1 -> [Pos_Motor_3_qc]
  Pos_Motor_4_qc/1 -> [Pos_Motor_4_qc]
  Output Value at Neutral Position3/1 -> Minus2/2
  threshold/1 -> MATLAB Function1/2(threshold)
  MATLAB Function1/1(y) -> Minus2/1
  [Pos_IncreaseDecrease] -> MATLAB Function1/1(u)
  Minus2/1 -> Gain4/1
  [flag_change] -> Compare To Constant1/1
  Compare To Constant2/1 -> AND1/1
  Compare To Constant1/1 -> AND1/2
  [flag] -> Compare To Constant2/1
  AND1/1 -> [reset]
  Memory1/1 -> MATLAB Function4/1(otpt_last)
  [reset] -> MATLAB Function4/2(reset)
  MATLAB Function4/1(y) -> Scope4/1, Memory1/1, [Motor4_pos_Adjust_qc]  "Motor4_pos_Adjust_qc"

== system SoRo_Compliant_Demo_0906/Tension_Mode_flag=2/Subsystem ==
  tension_in : Inport
  position_in : Inport  Port=2
  Enable : EnablePort
  tension_out : Outport
  position_out : Outport  Port=2
  wires:
  tension_in/1 -> tension_out/1
  position_in/1 -> position_out/1

== system SoRo_Compliant_Demo_0906/Tension_Mode_flag=2/Subsystem1 ==
  tension_in : Inport
  position_in : Inport  Port=2
  Enable : EnablePort
  tension_out : Outport
  position_out : Outport  Port=2
  wires:
  tension_in/1 -> tension_out/1
  position_in/1 -> position_out/1
